simulink model "MSX60_10_PS"  (Simulink 7.9)
settings: Solver=ode14x  StartTime=0.0  StopTime=220  FixedStep=0.05  RelTol=1e-4
values from neighbouring files (symbols this model uses):
  n = 1.3    [MSX60DS.m]    (also in MSX60_10_RL.m; MSX60_10_by2_with_PandO.m; MSX60_10_by2_with_PandO_PS.m; MSX60_10_by2_with_PandO_US (1).m)
  Ns = 1    [MSX60DS.m]    (also in MSX60_10_RL.m; MSX60_10_by2_with_PandO.m; MSX60_10_by2_with_PandO_PS.m; MSX60_10_by2_with_PandO_US (1).m)
  Rs = 0.58    [MSX60DS.m]    (also in MSX60_10_RL.m; MSX60_10_by2_with_PandO.m; MSX60_10_by2_with_PandO_PS.m; MSX60_10_by2_with_PandO_US (1).m)
  Voc = Voc(1)    [MSX60DS.m]    (also in MSX60_10_RL.m = 21.1; MSX60_10_by2_with_PandO.m = 21.1; MSX60_10_by2_with_PandO_PS.m = 21.1; MSX60_10_by2_with_PandO_US (1).m = 21.1)
libraries: elec_lib x10, nesl_utility x6, fl_lib x3, simulink x1
settings Model: Creator=pc1  LastModifiedBy=pc1
settings SolverCC: SolverJacobianMethodControl=SparsePerturbation
settings DataIOCC: SaveState=on

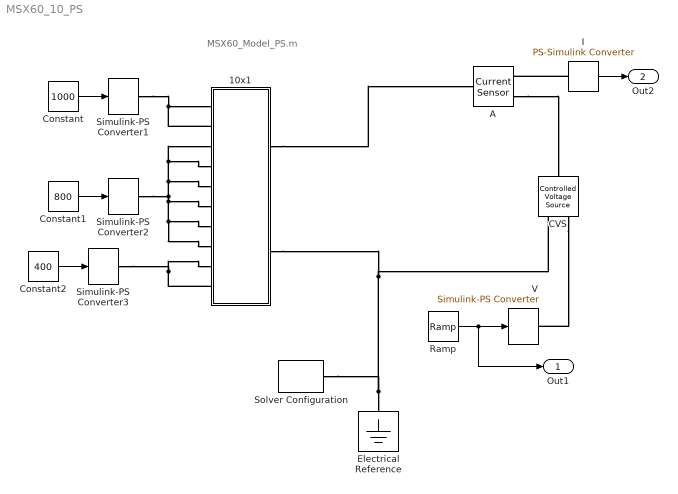
== system MSX60_10_PS ==
  note: MSX60_Model_PS.m
  10x1 : Subsystem
  A : fl_lib/Electrical/Electrical Sensors/Current Sensor  i1_Log=off  v1_Log=off  LocalVarNames=|i1|v1  LocalVarDescs=|i1|v1  LocalVarLogging=[0 0]
  CVS : fl_lib/Electrical/Electrical Sources/Controlled Voltage Source  i_Log=off  v_Log=off  LocalVarNames=|i|v  LocalVarDescs=|i|v  LocalVarLogging=[0 0]
  Constant : Constant  Value=1000
  Constant1 : Constant  Value=800
  Constant2 : Constant  Value=400
  Electrical Reference : fl_lib/Electrical/Electrical Elements/Electrical Reference  i_Log=off  LocalVarNames=|i  LocalVarDescs=|i  LocalVarLogging=0
  I : nesl_utility/PS-Simulink Converter  PhysicalDomain=network_engine_domain  LeftPortType=input  RightPortType=output  SubClassName=ps_output  Unit=1  AffineConversion=off
  Ramp : simulink/Sources/Ramp  slope=1  start=1  X0=0
  Simulink-PS Converter1 : nesl_utility/Simulink-PS Converter  PhysicalDomain=network_engine_domain  LeftPortType=input  RightPortType=output  SubClassName=ps_input  Unit=1  AffineConversion=off  InputFilterTimeConstant=.001  UdotUserProvided=[]  SimscapeFilterOrder=1  InputFiltering=off
  Simulink-PS Converter2 : nesl_utility/Simulink-PS Converter  PhysicalDomain=network_engine_domain  LeftPortType=input  RightPortType=output  SubClassName=ps_input  Unit=1  AffineConversion=off  InputFilterTimeConstant=.001  UdotUserProvided=[]  SimscapeFilterOrder=1  InputFiltering=off
  Simulink-PS Converter3 : nesl_utility/Simulink-PS Converter  PhysicalDomain=network_engine_domain  LeftPortType=input  RightPortType=output  SubClassName=ps_input  Unit=1  AffineConversion=off  InputFilterTimeConstant=.001  UdotUserProvided=[]  SimscapeFilterOrder=1  InputFiltering=off
  Solver Configuration : nesl_utility/Solver Configuration  PhysicalDomain=network_engine_domain  LeftPortType=input  RightPortType=generic  SubClassName=solver  UseCustomDae=off  DoDC=on  ResidualTolerance=1e-9  UseLocalSolver=off  LocalSolverChoice=NE_BACKWARD_EULER_ADVANCER  LocalSolverSampleTime=.001  DoFixedCost=off  MaxNonlinIter=3  MaxModeIter=2  LinearAlgebra=Sparse  Accelerate=off  Profile=off  UseLocalSampling=off  DelaysMemoryBudget=1024
  V : nesl_utility/Simulink-PS Converter  PhysicalDomain=network_engine_domain  LeftPortType=input  RightPortType=output  SubClassName=ps_input  Unit=1  AffineConversion=off  InputFilterTimeConstant=.001  UdotUserProvided=[]  SimscapeFilterOrder=1  InputFiltering=off
  Out1 : Outport
  Out2 : Outport  Port=2
  wires:
  Ramp/1 -> V/1, Out1/1
  I/1 -> Out2/1
  Constant/1 -> Simulink-PS Converter1/1
  Constant1/1 -> Simulink-PS Converter2/1
  Constant2/1 -> Simulink-PS Converter3/1
  connections:
  Electrical Reference/LConn1 -- Solver Configuration/RConn1 -- CVS/RConn2 -- 10x1/RConn2
  A/RConn2 -- CVS/LConn1
  CVS/RConn1 -- V/RConn1
  I/LConn1 -- A/RConn1
  10x1/LConn2 -- 10x1/LConn1 -- Simulink-PS Converter1/RConn1
  10x1/LConn6 -- 10x1/LConn7 -- 10x1/LConn8 -- 10x1/LConn5 -- 10x1/LConn4 -- 10x1/LConn3 -- Simulink-PS Converter2/RConn1
  10x1/LConn10 -- 10x1/LConn9 -- Simulink-PS Converter3/RConn1
  10x1/RConn1 -- A/LConn1

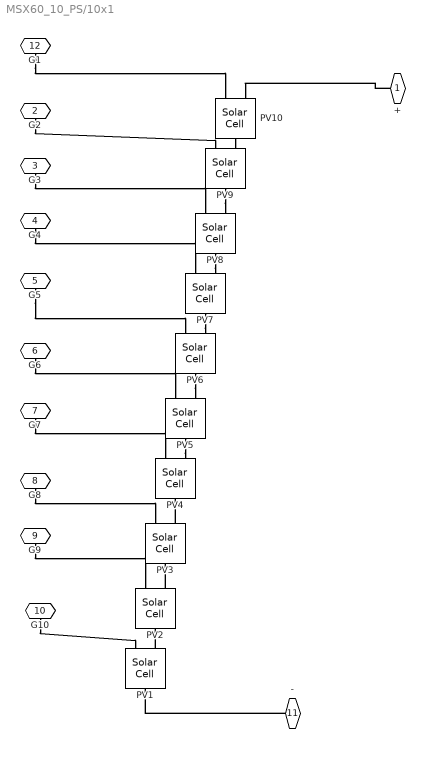
== system MSX60_10_PS/10x1 ==
  PV{1..10} (10 alike) : elec_lib/Sources/Solar Cell  prm=1  Isc=Isc A  Voc=Voc*Ns V  Is=1e-6 A  Is2=0 A  Iph=3.8 A  Ir0=Gstc W/m^2  ec=n*Voc*Ns  N2=0  Rs=Rs*Ns Ohm  Rp=Inf Ohm  TIPH1=0 1/K  EG=1.11 eV  TXIS1=3  TXIS2=3  TRS1=0  TRP1=0  Tmeas=25 C  TFIXED=25 C  LocalVarLogging=[]  thermal_mass=100 J/K  initial_temperature=25 C
  + : PMIOPort  Port=1  Side=Right
  G2 : PMIOPort  Port=2  Side=Left
  G3 : PMIOPort  Port=3  Side=Left
  G4 : PMIOPort  Port=4  Side=Left
  G5 : PMIOPort  Port=5  Side=Left
  G6 : PMIOPort  Port=6  Side=Left
  G7 : PMIOPort  Port=7  Side=Left
  G8 : PMIOPort  Port=8  Side=Left
  G9 : PMIOPort  Port=9  Side=Left
  G10 : PMIOPort  Port=10  Side=Left
  - : PMIOPort  Port=11  Side=Right
  G1 : PMIOPort  Port=12  Side=Left
  connections:
  PV1/LConn2 -- PV2/RConn1
  PV10/RConn1 -- PV9/LConn2
  PV2/LConn2 -- PV3/RConn1
  PV3/LConn2 -- PV4/RConn1
  PV5/RConn1 -- PV4/LConn2
  PV6/RConn1 -- PV5/LConn2
  PV7/RConn1 -- PV6/LConn2
  PV8/RConn1 -- PV7/LConn2
  PV9/RConn1 -- PV8/LConn2
  +/RConn1 -- PV10/LConn2
  G2/RConn1 -- PV9/LConn1
  G3/RConn1 -- PV8/LConn1
  G4/RConn1 -- PV7/LConn1
  G5/RConn1 -- PV6/LConn1
  G6/RConn1 -- PV5/LConn1
  G7/RConn1 -- PV4/LConn1
  G8/RConn1 -- PV3/LConn1
  G9/RConn1 -- PV2/LConn1
  G10/RConn1 -- PV1/LConn1
  -/RConn1 -- PV1/RConn1
  G1/RConn1 -- PV10/LConn1
